simulink model "system_model"  (R2022b)
settings: Solver=VariableStepAuto  StartTime=0.0  StopTime=10.0  RelTol=1e-3
libraries: prociolib x2
settings Model: Creator=vaz17  LastModifiedBy=zavic

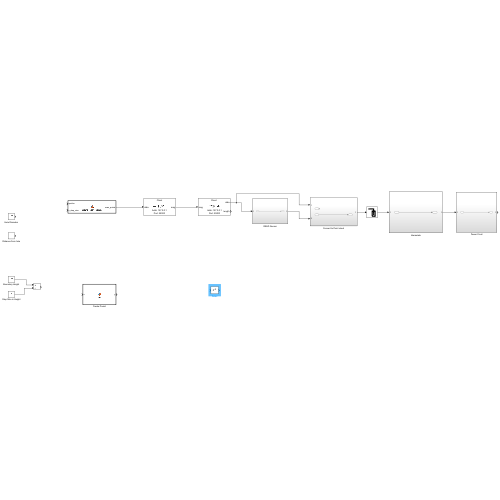
[thumbnail: Simulink's stored preview of the top-level diagram]
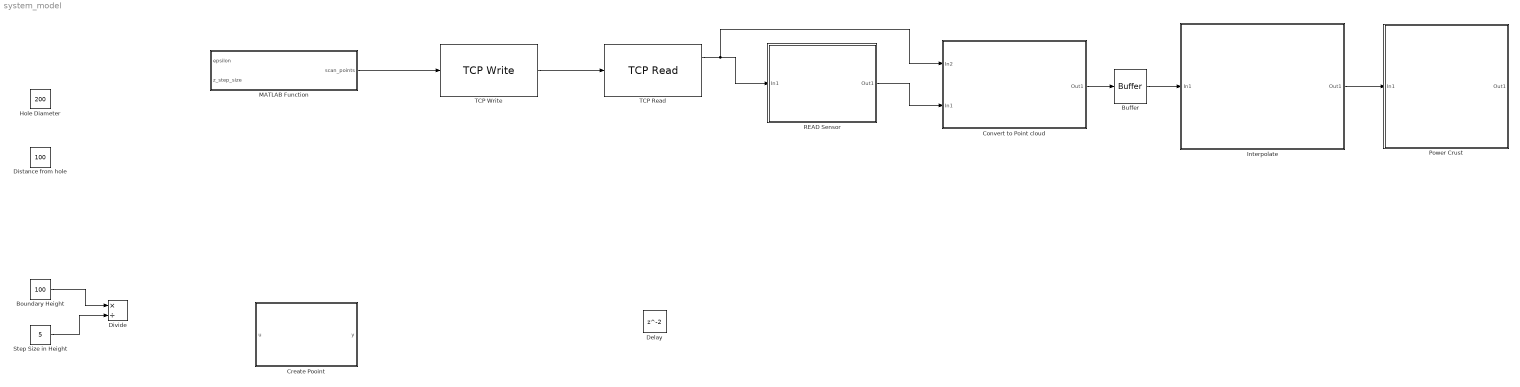
== system system_model ==
  Boundary Height : Constant  Value=100
  Buffer : Buffer  OutputFrames=off
  Convert to Point cloud : Subsystem
  Create Pooint : MATLAB Function  TreatAsAtomicUnit=on
  Delay : Delay
  Distance from hole : Constant  Value=100
  Divide : Product  Inputs=*/
  Hole Diameter : Constant  Value=200
  Interpolate : Subsystem
  MATLAB Function : MATLAB Function  TreatAsAtomicUnit=on
  Power Crust : Subsystem
  READ Sensor : Subsystem
  Step Size in Height : Constant  Value=5
  TCP Read : prociolib/TCP Read  NetworkRole=Client  RemoteAddress=127.0.0.1  RemotePort=25000  LocalPort=-1  DataType=uint8  DataLength=1  ByteOrder=LittleEndian  EnableEvent=off  OutputVarSizeSignal=off  OutputStatus=off  SampleTime=-1  hoistedMaskSrc=Variant/CODEGEN/TCP Read
  TCP Write : prociolib/TCP Write  NetworkRole=Client  RemoteAddress=127.0.0.1  RemotePort=25000  LocalPort=-1  ByteOrder=LittleEndian  OutputStatus=off  hoistedMaskSrc=Variant/CODEGEN/TCP Write
  wires:
  MATLAB Function/1(scan_points) -> TCP Write/1
  TCP Write/1 -> TCP Read/1
  TCP Read/1 -> Convert to Point cloud/1(In2), READ Sensor/1(In1)
  READ Sensor/1(Out1) -> Convert to Point cloud/2(In1)
  Convert to Point cloud/1(Out1) -> Buffer/1
  Buffer/1 -> Interpolate/1(In1)
  Interpolate/1(Out1) -> Power Crust/1(In1)
  Boundary Height/1 -> Divide/1
  Step Size in Height/1 -> Divide/2

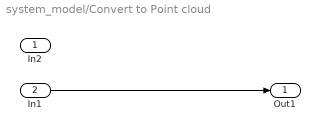
== system system_model/Convert to Point cloud ==
  In2 : Inport
  In1 : Inport  Port=2
  Out1 : Outport
  wires:
  In1/1 -> Out1/1

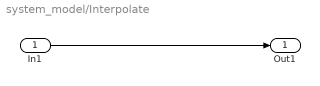
== system system_model/Interpolate ==
  In1 : Inport
  Out1 : Outport
  wires:
  In1/1 -> Out1/1

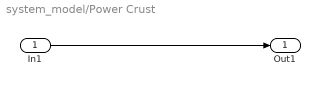
== system system_model/Power Crust ==
  In1 : Inport
  Out1 : Outport
  wires:
  In1/1 -> Out1/1

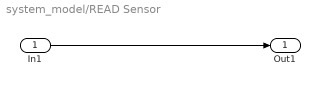
== system system_model/READ Sensor ==
  In1 : Inport
  Out1 : Outport
  wires:
  In1/1 -> Out1/1

== matlab function system_model/MATLAB Function ==
  data: epsilon input; scan_points output; z_step_size input
function scan_points = create_scan_points(epsilon,z_step_size)
%CREATE_SCAN_POINTS Summary of this function goes here
%   Detailed explanation goes here

hole_diameter = 200 ; %CM 

% it assumes a cylindrical boundary box arround the table hole. 
% The cylindrical boundary center matches the hole in the table and have
% the same diameter. 
% The maximum heigh is assumed to be 20 cm 
boundary_height = 200;


num_z_step = (boundary_height)/(z_step_size); % number of steps 

% Z of all scanning heights
Z = linspace(0,-boundary_height, num_z_step+1);

% Make it better later
azimuth = (pi.*linspace(0,360-18,21))./180 ;

R_epsi = hole_diameter/2 + epsilon;

scan_points = [];

for i = 1:length(azimuth)
 
    for j = 1 :length(Z)
        % Create coordinate in base space
        point_c_space(:,1) = R_epsi.*cos(azimuth(i));
        point_c_space(:,2) = R_epsi.*sin(azimuth(i));
        point_c_space(:,3) = Z(j);

        % Create Homogeneous Transformations with orientation
        HT = se3(roty(90)*rotx(azimuth(i)),point_c_space);
        
        % Convert to position and roll pith yaw
        scan_pos = [HT.trvec, tform2eul(HT.tform)];

        scan_points = [scan_points;scan_pos];
    end

end


end

== matlab function system_model/Create Pooint ==
  data: u input; y output
function y = fcn(u)

y = u;
